simulink subsystem "acceleration"  (R2021a)
settings: Solver=VariableStepAuto  StartTime=0.0  StopTime=10.0  RelTol=1e-3
settings Model: Creator=SeverinBeger  LastModifiedBy=SeverinBeger

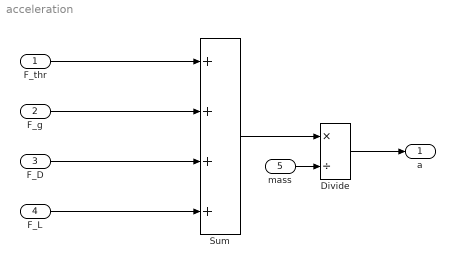
== system acceleration ==
  F_thr : Inport
  F_g : Inport  Port=2
  F_D : Inport  Port=3
  F_L : Inport  Port=4
  mass : Inport  Port=5
  Divide : Product  Inputs=*/
  Sum : Sum  Inputs=++++
  a : Outport
  wires:
  Sum/1 -> Divide/1
  F_D/1 -> Sum/3
  mass/1 -> Divide/2
  F_g/1 -> Sum/2
  F_thr/1 -> Sum/1
  Divide/1 -> a/1
  F_L/1 -> Sum/4
